simulink model "Q3sim4"  (R2022a)
settings: Solver=VariableStepAuto  StartTime=0.0  StopTime=8  RelTol=1e-6
values from neighbouring files (symbols this model uses):
  A = [zeros(4,1) A]    [Q3.m]
  B = B(:,1)    [Q3.m]
  Dsim = [zeros(4,1)]    [Q3.m]
  x0 = [0 0 pi/4 0]    [Q3.m]
settings Model: Creator=Crippa  LastModifiedBy=Crippa
settings SolverCC: ZeroCrossControl=DisableAll

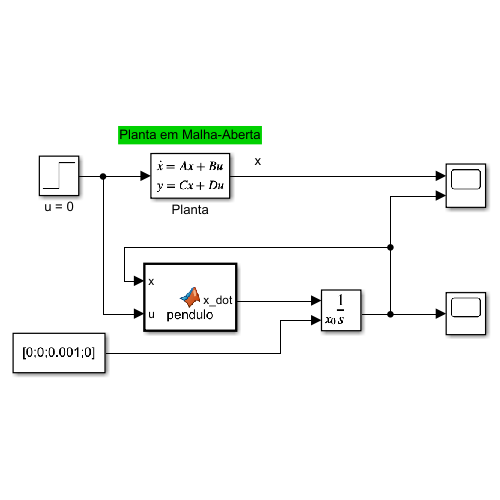
[thumbnail: Simulink's stored preview of the top-level diagram]
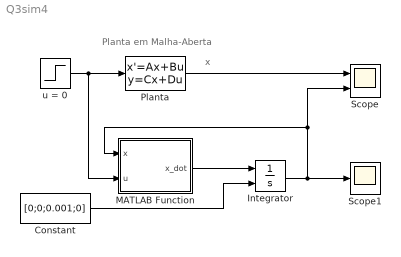
== system Q3sim4 ==
  note: x
  note: Planta em Malha-Aberta
  Constant : Constant  Value=[0;0;0.001;0]  VectorParams1D=off
  Integrator : Integrator  InitialConditionSource=external
  MATLAB Function : MATLAB Function  TreatAsAtomicUnit=on
  Planta : StateSpace  A=A  B=B  C=eye(4)  D=Dsim  InitialCondition=x0
  Scope : Scope  NumInputPorts=2
  Scope1 : Scope
  u = 0 : Step  Time=0  After=0  SampleTime=0
  wires:
  u = 0/1 -> MATLAB Function/2(u), Planta/1
  Planta/1 -> Scope/1
  MATLAB Function/1(x_dot) -> Integrator/1
  Integrator/1 -> Scope/2, MATLAB Function/1(x), Scope1/1
  Constant/1 -> Integrator/2

== matlab function Q3sim4/MATLAB Function ==
  data: x input; u input; x_dot output
function x_dot = pendulo(x,u)
    % x1 = y, x2 = y', x3 = theta, x4 = theta'

    % Parâmetros do pêndulo invertido
    M = 1; 
    m = 0.5;
    L = 1; 
    g = 9.81;

    x1 = x(1);
    x2 = x(2);
    x3 = x(3);
    x4 = x(4);

    % Dinâmica dos estados
    f1 = x2;
    f2 = (-m*g*sin(x3)*cos(x3) + m*L*(x4^2)*sin(x3)) / (M+m-m*cos(x3)^2);
    f3 = x4;
    f4 = g*sin(x3)/L - f2*cos(x3)/L;
    
    % Dinâmica do controle
    g1 = 0;
    g2 = u/(M+m-m*cos(x3)^2);
    g3 = 0;
    g4 = -cos(x3)/L * u/(M+m-m*cos(x3)^2);
    
    f = [f1; f2; f3; f4];
    g = [g1; g2; g3; g4];

    x_dot = f + g;
end
